simulink model "Synch_Machine_Simple"  (R2014a)
settings: Solver=ode23tb  StartTime=0.0  StopTime=10  RelTol=1e-3
PostLoadFcn:
  | warning off Simulink:Engine:UsingDefaultMaxStepSize
libraries: powerlib x4
Description:
  | Copyright 2014 The MathWorks, Inc.
settings Model: Creator=smiller  LastModifiedBy=psanghvi
settings DebuggingCC: UnderspecifiedInitializationDetection=Classic  StateNameClashWarn=warning

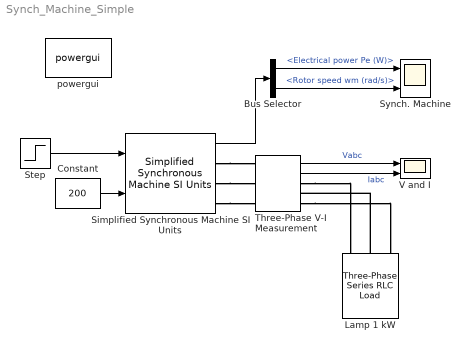
== system Synch_Machine_Simple ==
  Bus Selector : BusSelector  OutputSignals=Electrical power Pe (W),Rotor speed wm (rad/s)
  Constant : Constant  Value=200
  Lamp 1 kW : powerlib/Elements/Three-Phase Series RLC Load  LConnTagsString=A|B|C  Configuration=Y (grounded)  NominalVoltage=(200)*1  NominalFrequency=400  ActivePower=1e3  InductivePower=0  CapacitivePower=0  Measurements=None  LoadType=constant PQ
  Simplified Synchronous Machine SI Units : powerlib/Machines/Simplified Synchronous Machine SI Units  ConnectionType=3-wire Y  MechanicalLoad=Mechanical power Pm  MeasurementBus=off  NominalParameters=[50e3 200 400]  Mechanical="[0.2,  10,  2]"  InternalRL="[0.0204  0.8104e-3]"  InitialConditions=[0 0 0 0 0 0 0 0]  Units=1  LoadFlowParameters=[1 0 0 0 0]  TsPowergui=0  TsBlock=-1  BusType=swing  Pref=0  Qref=0  Qmin=-inf  Qmax=+inf  PLF=0  QLF=0
  Step : Step  Time=5  After=50e3  SampleTime=0
  Synch. Machine : Scope  NumInputPorts=2
      settings: TimeRange=10  YMin=0~1250  YMax=1000~1400
  Three-Phase V-I Measurement : powerlib/Measurements/Three-Phase V-I Measurement  VoltageMeasurement=phase-to-ground  SetLabelV=off  LabelV=Vabc  Vpu=off  VpuLL=off  CurrentMeasurement=yes  SetLabelI=off  LabelI=Iabc  Ipu=off  Pbase=100e6  Vbase=500e3  OutputType=Complex  PhasorSimulation=off  PSBequivalent=0
  V and I : Scope  NumInputPorts=2
      settings: TimeRange=0.01  YMin=-200~-5  YMax=200~5
  powergui : powerlib/powergui  Priority=1  SimulationMode=Continuous  SolverType=Tustin  SampleTime=50e-6  frequency=60  SPID=off  DisableSnubberDevices=off  DisableRonSwitches=off  DisableVfSwitches=off  SwTol=0  Interpol=off  DisplayEquations=off  Ts=0  methode=off  frequencyindice=400  Pbase=100e6  ErrMax=0.0001  Iterations=50  UnitsV=kV  UnitsW=MW  FunctionMessages=off  echomessages=off  HookPort=off  EnableUseOfTLC=off  x0status=blocks  RestoreLinks=warning  ResistiveCurrentMeasurement=off  Frange=[0:2:500]  Ylog=off  Xlog=on  ShowGrid=off  save=off  variable=ZData  structure=0  ZoomFFT=off  StartTime=0.0  cycles=1  DisplayStyle=1  fundamental=60  FreqAxis=off  MaxFrequency=1000  frequencyindicesteady=1  RmsSteady=1  display=off
  wires:
  Constant/1 -> Simplified Synchronous Machine SI Units/2
  Step/1 -> Simplified Synchronous Machine SI Units/1
  Simplified Synchronous Machine SI Units/1 -> Bus Selector/1
  Bus Selector/2 -> Synch. Machine/2  "<Rotor speed wm (rad/s)>"
  Bus Selector/1 -> Synch. Machine/1  "<Electrical power Pe (W)>"
  Three-Phase V-I Measurement/1 -> V and I/1  "Vabc"
  Three-Phase V-I Measurement/2 -> V and I/2  "Iabc"
  connections:
  Simplified Synchronous Machine SI Units/RConn2 -- Three-Phase V-I Measurement/LConn2
  Simplified Synchronous Machine SI Units/RConn1 -- Three-Phase V-I Measurement/LConn1
  Simplified Synchronous Machine SI Units/RConn3 -- Three-Phase V-I Measurement/LConn3
  Three-Phase V-I Measurement/RConn1 -- Lamp 1 kW/LConn1
  Lamp 1 kW/LConn2 -- Three-Phase V-I Measurement/RConn2
  Three-Phase V-I Measurement/RConn3 -- Lamp 1 kW/LConn3
